simulink library "MSM_element"  (R2023b)
settings: Solver=VariableStepAuto  StartTime=0.0  StopTime=10.0  RelTol=1e-3
values from neighbouring files (symbols this model uses):
  A0 = msm_width * msm_height    (= 2.5e-06)    [MSM_mechanism_simulation_properties.m]    (also in MSM_simulation_data_processing.m = 4)
  constant_magnetic_stress = 3.27e+6    (= 3270000)    [MSM_mechanism_simulation_properties.m]
  contraction_initial = -msm_length * e_initial    (= -0.001)    [MSM_mechanism_simulation_properties.m]
  cos_a = cos(deg2rad(43.23))    [MSM_mechanism_simulation_properties.m]
  coulomb_friction_ts = 1e-10    [MSM_mechanism_simulation_properties.m]
  crystal_visualization_length = msm_length    (= 0.02)    [MSM_mechanism_simulation_properties.m]
  e_0 = 0.06    [MSM_mechanism_simulation_properties.m]
  k_0 = 11.8    [MSM_mechanism_simulation_properties.m]
  msm_height = 1e-3    (= 0.001)    [MSM_mechanism_simulation_properties.m]
  msm_length = 20e-3    (= 0.02)    [MSM_mechanism_simulation_properties.m]
  msm_mass = ro * A0 * msm_length    (= 0.0004)    [MSM_mechanism_simulation_properties.m]
  msm_width = 2.5e-3    (= 0.0025)    [MSM_mechanism_simulation_properties.m]    (also in model_validation.m = 0.001)
  one_side_absolute_offset = one_side_elongation_capacity * msm_length    (= 0.0001)    [MSM_mechanism_simulation_properties.m]
  ro = 8000    [MSM_mechanism_simulation_properties.m]
  tooth_pitch = tooth_pitch * tooth_size_modifier    (= 0.00039)    [MSM_mechanism_simulation_properties.m]    (also in get_tooth_properties.m = 0.00024661; msm_sim_runs_for_pid.m = evalin('base','tooth_pitch'); save_sim_result.m = evalin('base','tooth_pitch'))
  tooth_plate_height = 4.64e-3    (= 0.00464)    [MSM_mechanism_simulation_properties.m]
  Z = griddata(x,y,z,X,Y)    [MSM_simulation_data_processing.m]
undefined symbols (not defined in the file or in its folder): X, Y
libraries: sm_lib x14, nesl_utility x7, fl_lib x4
settings Model: Creator=h19343  LastModifiedBy=h19343
settings OptimizationCC: ReuseModelBlockBuffer=off

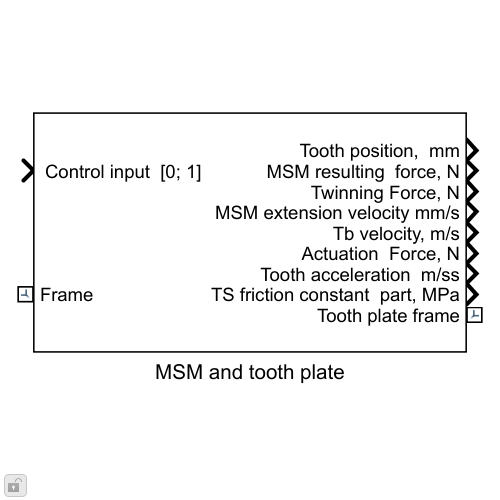
[thumbnail: Simulink's stored preview of the top-level diagram]
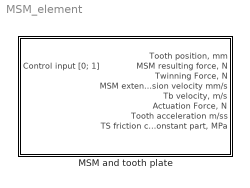
== system MSM_element ==
  MSM and tooth plate : Subsystem  mask{PositionTargetValue=contraction_initial}
      mask prompts: PositionTargetValue "ToothInitialPosition"
      mask TypeOptions PositionTargetValue: /PositionTargetValue

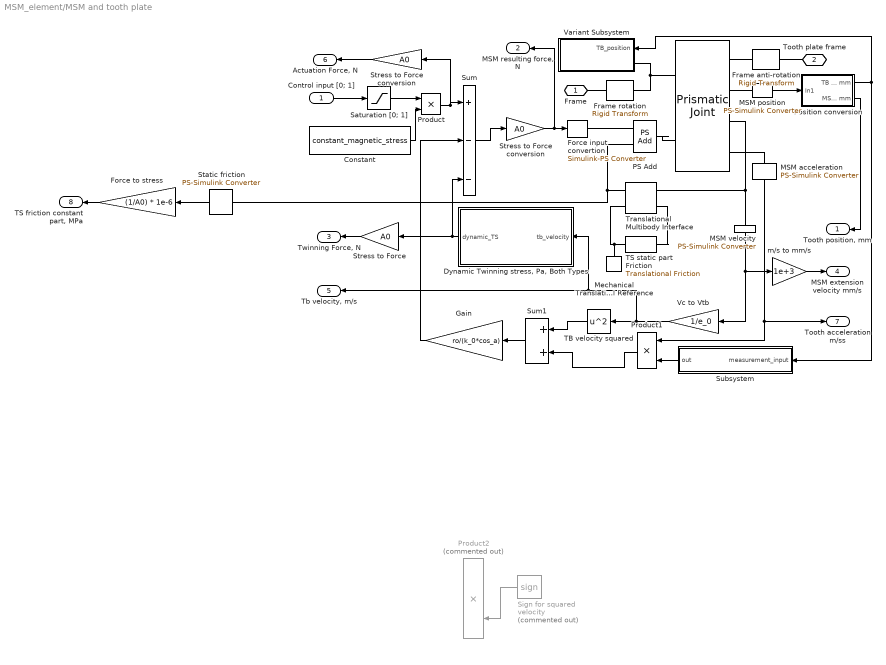
== system MSM_element/MSM and tooth plate ==
  " Control input [0; 1]" : Inport
  "   " : sm_lib/Joints/Prismatic Joint  JointMode=Normal  SenseConstraintForce=off  SenseConstraintForceX=off  SenseConstraintForceY=off  SenseConstraintForceZ=off  SenseConstraintTorque=off  SenseConstraintTorqueX=off  SenseConstraintTorqueY=off  SenseConstraintTorqueZ=off  SenseTotalForce=off  SenseTotalForceX=off  SenseTotalForceY=off  SenseTotalForceZ=off  SenseTotalTorque=off  SenseTotalTorqueX=off  SenseTotalTorqueY=off  SenseTotalTorqueZ=off  CompositeWrenchDir=FollowerOnBase  CompositeWrenchFrame=BaseFrame  EquilibriumPosition=0  EquilibriumPositionUnits=m  SpringStiffness=0  SpringStiffnessUnits=N/m  DampingCoefficient=bronze_steel_kinetic_friction  DampingCoefficientUnits=N/(m/s)  TorqueActuationMode=InputTorque  MotionActuationMode=ComputedMotion  SensePosition=on  SenseVelocity=on  SenseAcceleration=on  SenseTorqueForce=off  SenseLowerLimitTorqueForce=off  SenseUpperLimitTorqueForce=off  LowerLimitSpecify=on  LowerLimitBound=min_tooth_motion_range  LowerLimitBoundUnits=m  LowerLimitStiffness=1e6  LowerLimitStiffnessUnits=N/m  LowerLimitDamping=1e3  LowerLimitDampingUnits=N/(m/s)  LowerLimitTransitionRegionWidth=1e-4  LowerLimitTransitionRegionWidthUnits=m  UpperLimitSpecify=on  UpperLimitBound=max_tooth_motion_range  UpperLimitBoundUnits=m  UpperLimitStiffness=1e12  UpperLimitStiffnessUnits=N/m  UpperLimitDamping=1e4  UpperLimitDampingUnits=N/(m/s)  UpperLimitTransitionRegionWidth=1e-4  UpperLimitTransitionRegionWidthUnits=m  PositionTargetSpecify=on  PositionTargetPriority=Low  PositionTargetValue=PositionTargetValue  PositionTargetValueUnits=m  VelocityTargetSpecify=off  VelocityTargetPriority=High  VelocityTargetValue=0  VelocityTargetValueUnits=m/s
  Constant : Constant  Value=constant_magnetic_stress
  "Dynamic Twinning stress, Pa, Both Types" : MATLAB Function  TreatAsAtomicUnit=on
  Force input convertion : nesl_utility/Simulink-PS Converter  PhysicalDomain=network_engine_domain  SubClassName=ps_input  LeftPortType=input  RightPortType=output  PseudoPeriodic=off  Frequencies=[]  NoiseDistribution=none  NoiseParameters=[]  Unit=N  AffineConversion=off  FilteringAndDerivatives=filter  SimscapeFilterOrder=2  InputFilterTimeConstant=filter_time_constant  UdotUserProvided=0
  "Force to stress  " : Gain  Gain=(1/A0) * 1e-6
  Frame anti-rotation : sm_lib/Frames and Transforms/Rigid Transform  TranslationMethod=None  TranslationStandardOffset=0  TranslationStandardOffsetUnits=m  TranslationStandardAxis=+Z  TranslationCartesianOffset=[0 0 0]  TranslationCartesianOffsetUnits=m  TranslationROffset=0  TranslationROffsetUnits=m  TranslationZOffset=0  TranslationZOffsetUnits=m  TranslationThetaOffset=0  TranslationThetaOffsetUnits=deg  RotationMethod=StandardAxis  RotationAngleUnits=deg  RotationStandardAxis=-X  RotationAngle=-90  RotationArbitraryAxis=[0 0 1]  FollAlignAxisA=+X  BaseAlignAxisA=+Y  FollAlignAxisB=+Y  BaseAlignAxisB=+Z  RotationSequenceAxes=FollowerAxes  RotationSequence=XYX  RotationSequenceAngles=[0 0 0]  RotationSequenceAnglesUnits=deg  RotationMatrix=[1 0 0; 0 1 0; 0 0 1]  Quaternion=[1 0 0 0]
  Frame rotation : sm_lib/Frames and Transforms/Rigid Transform  TranslationMethod=None  TranslationStandardOffset=0  TranslationStandardOffsetUnits=m  TranslationStandardAxis=+Z  TranslationCartesianOffset=[0 0 0]  TranslationCartesianOffsetUnits=m  TranslationROffset=0  TranslationROffsetUnits=m  TranslationZOffset=0  TranslationZOffsetUnits=m  TranslationThetaOffset=0  TranslationThetaOffsetUnits=deg  RotationMethod=StandardAxis  RotationAngleUnits=deg  RotationStandardAxis=-X  RotationAngle=90  RotationArbitraryAxis=[0 0 1]  FollAlignAxisA=+X  BaseAlignAxisA=+Y  FollAlignAxisB=+Y  BaseAlignAxisB=+Z  RotationSequenceAxes=FollowerAxes  RotationSequence=XYX  RotationSequenceAngles=[0 0 0]  RotationSequenceAnglesUnits=deg  RotationMatrix=[1 0 0; 0 1 0; 0 0 1]  Quaternion=[1 0 0 0]
  Gain : Gain  Gain=ro/(k_0*cos_a)
  MSM acceleration : nesl_utility/PS-Simulink Converter  PhysicalDomain=network_engine_domain  SubClassName=ps_output  LeftPortType=input  RightPortType=output  PseudoPeriodic=off  Frequencies=[]  VectorFormat=inherit  Unit=inherit  AffineConversion=off
  MSM velocity : nesl_utility/PS-Simulink Converter  PhysicalDomain=network_engine_domain  SubClassName=ps_output  LeftPortType=input  RightPortType=output  PseudoPeriodic=off  Frequencies=[]  VectorFormat=inherit  Unit=inherit  AffineConversion=off
  MSM position : nesl_utility/PS-Simulink Converter  PhysicalDomain=network_engine_domain  SubClassName=ps_output  LeftPortType=input  RightPortType=output  PseudoPeriodic=off  Frequencies=[]  VectorFormat=inherit  Unit=inherit  AffineConversion=off
  Mechanical Translational Reference : fl_lib/Mechanical/Translational Elements/Mechanical Translational Reference
  PS Add : fl_lib/Physical Signals/Functions/PS Add
  Position conversion : Subsystem
  Product : Product
  Product1 : Product
  Product2 : Product  Commented=on
  Saturation [0; 1] : Saturate  UpperLimit=1  LowerLimit=0
  Sign for squared velocity : Signum  Commented=on
  Static friction : nesl_utility/PS-Simulink Converter  PhysicalDomain=network_engine_domain  SubClassName=ps_output  LeftPortType=input  RightPortType=output  PseudoPeriodic=off  Frequencies=[]  VectorFormat=inherit  Unit=inherit  AffineConversion=off
  Stress to Force : Gain  Gain=A0
  Stress to Force conversion : Gain  Gain=A0
  "Stress to Force conversion   " : Gain  Gain=A0
  Subsystem : Subsystem
      mask Display:
      | text(0.05,0.5,'{out =}  m_0 / ( \rho * A_0 ) + L - L_0',...
      | HorizontalAlignment = 'left',texmode = 'on')
  Sum : Sum  Inputs=+--
  Sum1 : Sum
  TB velocity squared : Math  Operator=square
  TS static part Friction : fl_lib/Mechanical/Translational Elements/Translational Friction  brkwy_frc=coulomb_friction_ts * (1 + 1e-5) N  brkwy_vel=1e-5 m/s  Col_frc=coulomb_friction_ts N  visc_coef=0 N*s/m  v_specify=off  v_priority=None  v=0 m/s  v_nominal_specify=off  v_nominal_unit=m/s  v_nominal_value=1  f_specify=off  f_priority=None  f=0 N  f_nominal_specify=off  f_nominal_unit=N  f_nominal_value=1
      settings: InternalSimscapePortConfiguration="{\"Bottom\":[],\"Left\":[{\"id\":\"R\",\"label\":\"R\",\"type\":\"foundation.mechanical.translational.translational\"}],\"Right\":[{\"id\":\"C\",\"label\":\"C\",\"type\":\"foundation.mechanical.translational.translational\"}],\"Top\":[]}"
  Translational Multibody Interface : fl_lib/Mechanical/Multibody Interfaces/Translational Multibody Interface
  Variant Subsystem : Subsystem  InitFcn=|  Variant=on
      | simple_visuals_variant = Simulink.Variant('simplified_visualization == true');
      | full_visuals_variant = Simulink.Variant('simplified_visualization == false');
      settings: PortSchema="{\"entries\":[{\"content\":{\"sides\":[{\"content\":{\"connectorIds\":[\"LConn1\",\"In1\"]},\"type\":\"ConnectorPlacement.EquallySpacedRectSide\",\"uuid\":\"521faf6a-dace-4634-9239-1a534469285d\"},{\"content\":{\"side\":\"RIGHT\"},\"type\":\"ConnectorPlacement.EquallySpacedRectSide\",\"uuid\":\"3bf57a7f-6223-4aa5-b9ce-2577a1bef6cc\"},{\"content\":{\"side\":\"TOP\"},\"type\":\"ConnectorPlacement.EquallySpacedRectSide\",\"uuid\":\"83854e2c-9733-4a76-abdf-07b6192acd72\"}]},\"type\":\"ConnectorPlacement.EquallySpacedConnector\",\"uuid\":\"3009cfd0-5b5f-49c0-93d8-2e0b9647e6c0\"}],\"packageUris\":[\"http://schema.mathworks.com/mf0/Connector/R2020b\"],\"version\":\"1.0\"}"
      mask Display:
      | text(0.05,0.65,'TB position',...
      | HorizontalAlignment = 'left',texmode = 'on')
      | text(0.05,0.35,'visualization block',...
      | HorizontalAlignment = 'left',texmode = 'on')
  Vc to Vtb : Gain  Gain=1/e_0
  m/s to mm/s : Gain  Gain=1e+3
  Frame : PMIOPort  Side=Left
  Tooth plate frame : PMIOPort  Port=2  Side=Right
  "Tooth position, mm" : Outport
  "      MSM resulting force, N" : Outport  Port=2
  "Twinning Force, N" : Outport  Port=3
  MSM extension velocity mm/s : Outport  Port=4
  "Tb velocity, m/s" : Outport  Port=5
  "Actuation Force, N" : Outport  Port=6
  Tooth acceleration m/ss : Outport  Port=7
  "TS friction constant part, MPa" : Outport  Port=8
  wires:
  " Control input [0; 1]"/1 -> Saturation [0; 1]/1
  Saturation [0; 1]/1 -> Product/1
  Constant/1 -> Product/2
  Stress to Force conversion/1 -> "      MSM resulting force, N"/1, Force input convertion/1
  Sum/1 -> Stress to Force conversion/1
  Product/1 -> Sum/1, "Stress to Force conversion   "/1
  Stress to Force/1 -> "Twinning Force, N"/1
  "Stress to Force conversion   "/1 -> "Actuation Force, N"/1
  MSM velocity/1 -> Vc to Vtb/1, m/s to mm/s/1
  "Dynamic Twinning stress, Pa, Both Types"/1(dynamic_TS) -> Sum/3, Stress to Force/1
  MSM acceleration/1 -> Tooth acceleration m/ss/1, Product1/1
  Sum1/1 -> Gain/1
  Product1/1 -> Sum1/2
  Sign for squared velocity/1 -> Product2/2
  Vc to Vtb/1 -> "Dynamic Twinning stress, Pa, Both Types"/1(tb_velocity), "Tb velocity, m/s"/1, TB velocity squared/1
  m/s to mm/s/1 -> MSM extension velocity mm/s/1
  "Force to stress  "/1 -> "TS friction constant part, MPa"/1
  TB velocity squared/1 -> Sum1/1
  Gain/1 -> Sum/2
  Subsystem/1(out) -> Product1/2
  Position conversion/1("TB pos, mm") -> Variant Subsystem/1(TB_position), Subsystem/1(measurement_input)
  MSM position/1 -> Position conversion/1(In1)
  Position conversion/2("MSM pos, mm") -> "Tooth position, mm"/1
  Static friction/1 -> "Force to stress  "/1
  connections:
  Tooth plate frame/RConn1 -- Frame anti-rotation/RConn1
  MSM position/LConn1 -- "   "/RConn2
  Frame anti-rotation/LConn1 -- "   "/RConn1
  "   "/LConn1 -- Frame rotation/RConn1 -- Variant Subsystem/LConn1
  Frame rotation/LConn1 -- Frame/RConn1
  Translational Multibody Interface/RConn1 -- MSM velocity/LConn1 -- "   "/RConn3
  MSM acceleration/LConn1 -- "   "/RConn4
  PS Add/LConn2 -- Translational Multibody Interface/LConn1 -- Static friction/LConn1
  Mechanical Translational Reference/LConn1 -- Translational Multibody Interface/LConn2 -- TS static part Friction/RConn1
  TS static part Friction/LConn1 -- Translational Multibody Interface/RConn2
  Force input convertion/RConn1 -- PS Add/LConn1
  PS Add/RConn1 -- "   "/LConn2

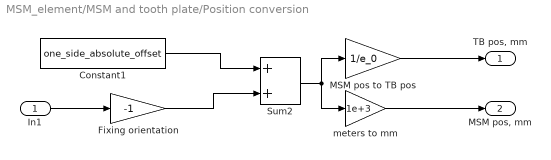
== system MSM_element/MSM and tooth plate/Position conversion ==
  In1 : Inport
  Constant1 : Constant  Value=one_side_absolute_offset
  Fixing orientation : Gain  Gain=-1
  MSM pos to TB pos : Gain  Gain=1/e_0
  Sum2 : Sum
  meters to mm : Gain  Gain=1e+3
  "TB pos, mm" : Outport
  "MSM pos, mm" : Outport  Port=2
  wires:
  Fixing orientation/1 -> Sum2/2
  Sum2/1 -> MSM pos to TB pos/1, meters to mm/1
  meters to mm/1 -> "MSM pos, mm"/1
  Constant1/1 -> Sum2/1
  In1/1 -> Fixing orientation/1
  MSM pos to TB pos/1 -> "TB pos, mm"/1

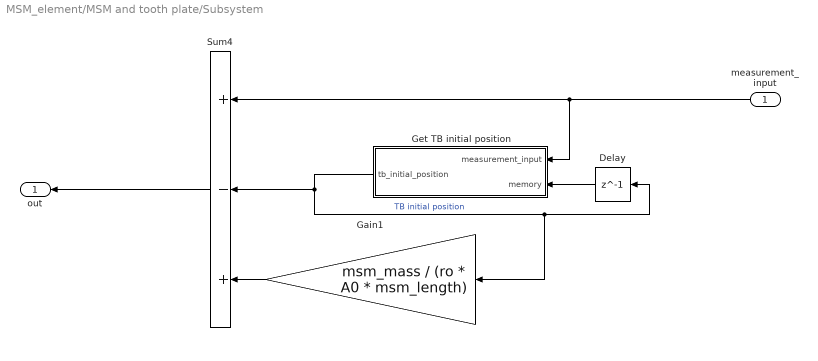
== system MSM_element/MSM and tooth plate/Subsystem ==
  measurement_input : Inport
  Delay : Delay  DelayLength=1  InitialCondition=-1
  Gain1 : Gain  Gain=msm_mass / (ro * A0 * msm_length)
  Get TB initial position : MATLAB Function  TreatAsAtomicUnit=on
  Sum4 : Sum  Inputs=+-+
  out : Outport
  wires:
  Get TB initial position/1(tb_initial_position) -> Gain1/1, Delay/1, Sum4/2  "TB initial position"
  Gain1/1 -> Sum4/3
  Delay/1 -> Get TB initial position/2(memory)
  measurement_input/1 -> Sum4/1, Get TB initial position/1(measurement_input)
  Sum4/1 -> out/1

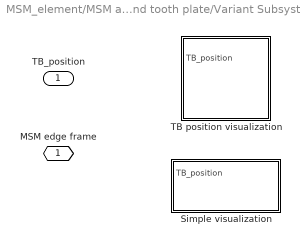
== system MSM_element/MSM and tooth plate/Variant Subsystem ==
  TB_position : Inport
  Simple visualization : Subsystem  VariantControl=simple_visuals_variant
  TB position visualization : Subsystem  AncestorBlock=MSM_element_08_04_2024/MSM and tooth plate/TB position visualization  VariantControl=full_visuals_variant
  MSM edge frame : PMIOPort  Side=Left

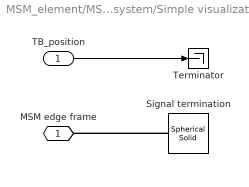
== system MSM_element/MSM and tooth plate/Variant Subsystem/Simple visualization ==
  TB_position : Inport
  Signal termination : sm_lib/Body Elements/Spherical Solid  GraphicAmbientColor=[0.15 0.15 0.15 1.0]  BasedOnType=Mass  CenterOfMass=[0 0 0]  CenterOfMassUnits=m  GraphicDiffuseColor=[0.5 0.5 0.5]  Density=1000  DensityUnits=kg/m^3  DoExposeReferenceFrame=on  GraphicEmissiveColor=[0.0 0.0 0.0 1.0]  ExportEntireGeometry=off  SerializedExposedGeometries=<ExposedGeometries/>  SerializedFrames=<Frames/>  MarkerShape=Sphere  MarkerSize=10  GraphicType=None  InertiaType=CalculateFromGeometry  Mass=1e-12  MassUnits=kg  MomentsOfInertia=[1 1 1]  MomentsOfInertiaUnits=kg*m^2  GraphicOpacity=1.0  ProductsOfInertia=[0 0 0]  ProductsOfInertiaUnits=kg*m^2  GraphicShininess=75  GraphicSpecularColor=[0.5 0.5 0.5 1.0]  SphereRadius=1  SphereRadiusUnits=m  GraphicVisPropType=SimpleVisualProperties
  Terminator : Terminator
  MSM edge frame : PMIOPort  Side=Left
  wires:
  TB_position/1 -> Terminator/1
  connections:
  Signal termination/RConn1 -- MSM edge frame/RConn1

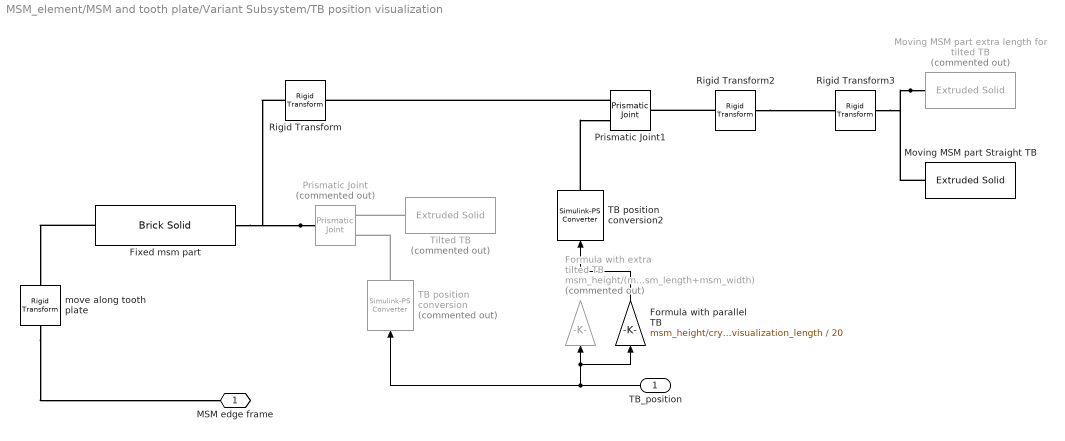
== system MSM_element/MSM and tooth plate/Variant Subsystem/TB position visualization ==
  TB_position : Inport
  Fixed msm part : sm_lib/Body Elements/Brick Solid  GraphicAmbientColor=[0.15 0.15 0.15 1.0]  BasedOnType=Mass  BrickDimensions=[msm_width msm_height crystal_visualization_length]  BrickDimensionsUnits=m  CenterOfMass=[0 0 0]  CenterOfMassUnits=m  GraphicDiffuseColor=[0.6 0.6 0.6]  Density=1000  DensityUnits=kg/m^3  DoExposeReferenceFrame=off  GraphicEmissiveColor=[0.0 0.0 0.0 1.0]  ExportEntireGeometry=off  SerializedFrames=<Frames><Frame><Id>Frame1</Id><Value><Name>End frame</Name><Origin><Source>GeometricFeature</Source><FeatureName>-z surface</FeatureName></Origin><PrimaryAxis><DefinedDirection>+Z</DefinedDirection><Source>ReferenceFrame</Source><SourceDirection>-Z</SourceDirection><FeatureName></FeatureName></PrimaryAxis><SecondaryAxis><DefinedDirection>+X</DefinedDirection><Source>ReferenceFrame</Source><SourceDirection>+X</SourceDirection><FeatureName></FeatureName></SecondaryAxis></Value></Frame><Frame><Id>Frame2</Id><Value><Name>End rotation</Name><Origin><Source>GeometricFeature</Source><FeatureName>+y -z curve</FeatureName></Origin><PrimaryAxis><DefinedDirection>+Z</DefinedDirection><Source>ReferenceFrame</Source><SourceDirection>-Z</SourceDirection><FeatureName></FeatureName></PrimaryAxis><SecondaryAxis><DefinedDirection>+X</DefinedDirection><Source>ReferenceFrame</Source><SourceDirection>+X</SourceDirection><FeatureName></FeatureName></SecondaryAxis></Value></Frame></Frames>  MarkerShape=Sphere  MarkerSize=10  GraphicType=FromGeometry  InertiaType=CalculateFromGeometry  Mass=1e-12  MassUnits=kg  MomentsOfInertia=[1 1 1]  MomentsOfInertiaUnits=kg*m^2  GraphicOpacity=1.0  ProductsOfInertia=[0 0 0]  ProductsOfInertiaUnits=kg*m^2  GraphicShininess=75  GraphicSpecularColor=[0.5 0.5 0.5 1.0]  GraphicVisPropType=SimpleVisualProperties
  Formula with extra tilted TB : Gain  Commented=on  Gain=msm_height/(msm_length+msm_width)
  Formula with parallel TB : Gain  Gain=msm_height/crystal_visualization_length / 20
  Moving MSM part Straight TB : sm_lib/Body Elements/Extruded Solid  GraphicAmbientColor=[0.15 0.15 0.15 1.0]  BasedOnType=Mass  CenterOfMass=[0 0 0]  CenterOfMassUnits=m  GraphicDiffuseColor=moving_tb_color  ExportConvexHullGeometry=off  ExtrusionCrossSection=[crystal_visualization_length msm_height / 20; 0 msm_height / 20; 0 0]  ExtrusionCrossSectionUnits=m  Density=1000  DensityUnits=kg/m^3  DoExposeReferenceFrame=on  GraphicEmissiveColor=[0.0 0.0 0.0 1.0]  ExportEntireGeometry=off  ExtrusionLength=msm_width  ExtrusionLengthUnits=m  ExtrusionType=General  SerializedFrames=<Frames/>  MarkerShape=Sphere  MarkerSize=10  GraphicType=FromGeometry  InertiaType=CalculateFromGeometry  Mass=1e-12  MassUnits=kg  MomentsOfInertia=[1 1 1]  MomentsOfInertiaUnits=kg*m^2  PolygonNumSides=3  GraphicOpacity=1.0  PolygonOuterRadius=1  PolygonOuterRadiusUnits=m  ProductsOfInertia=[0 0 0]  ProductsOfInertiaUnits=kg*m^2  GraphicShininess=75  GraphicSpecularColor=[0.5 0.5 0.5 1.0]  GraphicVisPropType=SimpleVisualProperties
  Moving MSM part extra length for tilted TB : sm_lib/Body Elements/Extruded Solid  Commented=on  GraphicAmbientColor=[0.15 0.15 0.15 1.0]  BasedOnType=Mass  CenterOfMass=[0 0 0]  CenterOfMassUnits=m  GraphicDiffuseColor=moving_tb_color  ExportConvexHullGeometry=off  ExtrusionCrossSection=[msm_length+msm_width msm_height; 0 msm_height; 0 0]  ExtrusionCrossSectionUnits=m  Density=1000  DensityUnits=kg/m^3  DoExposeReferenceFrame=on  GraphicEmissiveColor=[0.0 0.0 0.0 1.0]  ExportEntireGeometry=off  ExtrusionLength=msm_width  ExtrusionLengthUnits=m  ExtrusionType=General  SerializedFrames=<Frames/>  MarkerShape=Sphere  MarkerSize=10  GraphicType=FromGeometry  InertiaType=CalculateFromGeometry  Mass=1e-12  MassUnits=kg  MomentsOfInertia=[1 1 1]  MomentsOfInertiaUnits=kg*m^2  PolygonNumSides=3  GraphicOpacity=1.0  PolygonOuterRadius=1  PolygonOuterRadiusUnits=m  ProductsOfInertia=[0 0 0]  ProductsOfInertiaUnits=kg*m^2  GraphicShininess=75  GraphicSpecularColor=[0.5 0.5 0.5 1.0]  GraphicVisPropType=SimpleVisualProperties
  Prismatic Joint : sm_lib/Joints/Prismatic Joint  Commented=on  JointMode=Normal  SenseConstraintForce=off  SenseConstraintForceX=off  SenseConstraintForceY=off  SenseConstraintForceZ=off  SenseConstraintTorque=off  SenseConstraintTorqueX=off  SenseConstraintTorqueY=off  SenseConstraintTorqueZ=off  SenseTotalForce=off  SenseTotalForceX=off  SenseTotalForceY=off  SenseTotalForceZ=off  SenseTotalTorque=off  SenseTotalTorqueX=off  SenseTotalTorqueY=off  SenseTotalTorqueZ=off  CompositeWrenchDir=FollowerOnBase  CompositeWrenchFrame=BaseFrame  EquilibriumPosition=0  EquilibriumPositionUnits=m  SpringStiffness=0  SpringStiffnessUnits=N/m  DampingCoefficient=0  DampingCoefficientUnits=N/(m/s)  TorqueActuationMode=ComputedTorque  MotionActuationMode=InputMotion  SensePosition=off  SenseVelocity=off  SenseAcceleration=off  SenseTorqueForce=off  SenseLowerLimitTorqueForce=off  SenseUpperLimitTorqueForce=off  LowerLimitSpecify=off  LowerLimitBound=-1  LowerLimitBoundUnits=m  LowerLimitStiffness=1e6  LowerLimitStiffnessUnits=N/m  LowerLimitDamping=1e3  LowerLimitDampingUnits=N/(m/s)  LowerLimitTransitionRegionWidth=1e-4  LowerLimitTransitionRegionWidthUnits=m  UpperLimitSpecify=off  UpperLimitBound=1  UpperLimitBoundUnits=m  UpperLimitStiffness=1e6  UpperLimitStiffnessUnits=N/m  UpperLimitDamping=1e3  UpperLimitDampingUnits=N/(m/s)  UpperLimitTransitionRegionWidth=1e-4  UpperLimitTransitionRegionWidthUnits=m  PositionTargetSpecify=off  PositionTargetPriority=High  PositionTargetValue=0  PositionTargetValueUnits=m  VelocityTargetSpecify=off  VelocityTargetPriority=High  VelocityTargetValue=0  VelocityTargetValueUnits=m/s
  Prismatic Joint1 : sm_lib/Joints/Prismatic Joint  JointMode=Normal  SenseConstraintForce=off  SenseConstraintForceX=off  SenseConstraintForceY=off  SenseConstraintForceZ=off  SenseConstraintTorque=off  SenseConstraintTorqueX=off  SenseConstraintTorqueY=off  SenseConstraintTorqueZ=off  SenseTotalForce=off  SenseTotalForceX=off  SenseTotalForceY=off  SenseTotalForceZ=off  SenseTotalTorque=off  SenseTotalTorqueX=off  SenseTotalTorqueY=off  SenseTotalTorqueZ=off  CompositeWrenchDir=FollowerOnBase  CompositeWrenchFrame=BaseFrame  EquilibriumPosition=0  EquilibriumPositionUnits=m  SpringStiffness=0  SpringStiffnessUnits=N/m  DampingCoefficient=0  DampingCoefficientUnits=N/(m/s)  TorqueActuationMode=ComputedTorque  MotionActuationMode=InputMotion  SensePosition=off  SenseVelocity=off  SenseAcceleration=off  SenseTorqueForce=off  SenseLowerLimitTorqueForce=off  SenseUpperLimitTorqueForce=off  LowerLimitSpecify=off  LowerLimitBound=-1  LowerLimitBoundUnits=m  LowerLimitStiffness=1e6  LowerLimitStiffnessUnits=N/m  LowerLimitDamping=1e3  LowerLimitDampingUnits=N/(m/s)  LowerLimitTransitionRegionWidth=1e-4  LowerLimitTransitionRegionWidthUnits=m  UpperLimitSpecify=off  UpperLimitBound=1  UpperLimitBoundUnits=m  UpperLimitStiffness=1e6  UpperLimitStiffnessUnits=N/m  UpperLimitDamping=1e3  UpperLimitDampingUnits=N/(m/s)  UpperLimitTransitionRegionWidth=1e-4  UpperLimitTransitionRegionWidthUnits=m  PositionTargetSpecify=off  PositionTargetPriority=High  PositionTargetValue=0  PositionTargetValueUnits=m  VelocityTargetSpecify=off  VelocityTargetPriority=High  VelocityTargetValue=0  VelocityTargetValueUnits=m/s
  Rigid Transform : sm_lib/Frames and Transforms/Rigid Transform  TranslationMethod=None  TranslationStandardOffset=0  TranslationStandardOffsetUnits=m  TranslationStandardAxis=+Z  TranslationCartesianOffset=[0 0 0]  TranslationCartesianOffsetUnits=m  TranslationROffset=0  TranslationROffsetUnits=m  TranslationZOffset=0  TranslationZOffsetUnits=m  TranslationThetaOffset=0  TranslationThetaOffsetUnits=deg  RotationMethod=StandardAxis  RotationAngleUnits=deg  RotationStandardAxis=+X  RotationAngle=90  RotationArbitraryAxis=[0 0 1]  FollAlignAxisA=+X  BaseAlignAxisA=+Y  FollAlignAxisB=+Y  BaseAlignAxisB=+Z  RotationSequenceAxes=FollowerAxes  RotationSequence=XYX  RotationSequenceAngles=[0 0 0]  RotationSequenceAnglesUnits=deg  RotationMatrix=[1 0 0; 0 1 0; 0 0 1]  Quaternion=[1 0 0 0]
  Rigid Transform2 : sm_lib/Frames and Transforms/Rigid Transform  TranslationMethod=None  TranslationStandardOffset=0  TranslationStandardOffsetUnits=m  TranslationStandardAxis=+Z  TranslationCartesianOffset=[0 0 0]  TranslationCartesianOffsetUnits=m  TranslationROffset=0  TranslationROffsetUnits=m  TranslationZOffset=0  TranslationZOffsetUnits=m  TranslationThetaOffset=0  TranslationThetaOffsetUnits=deg  RotationMethod=StandardAxis  RotationAngleUnits=deg  RotationStandardAxis=+X  RotationAngle=90  RotationArbitraryAxis=[0 0 1]  FollAlignAxisA=+X  BaseAlignAxisA=+Y  FollAlignAxisB=+Y  BaseAlignAxisB=+Z  RotationSequenceAxes=FollowerAxes  RotationSequence=XYX  RotationSequenceAngles=[0 0 0]  RotationSequenceAnglesUnits=deg  RotationMatrix=[1 0 0; 0 1 0; 0 0 1]  Quaternion=[1 0 0 0]
  Rigid Transform3 : sm_lib/Frames and Transforms/Rigid Transform  TranslationMethod=None  TranslationStandardOffset=0  TranslationStandardOffsetUnits=m  TranslationStandardAxis=+Z  TranslationCartesianOffset=[0 0 0]  TranslationCartesianOffsetUnits=m  TranslationROffset=0  TranslationROffsetUnits=m  TranslationZOffset=0  TranslationZOffsetUnits=m  TranslationThetaOffset=0  TranslationThetaOffsetUnits=deg  RotationMethod=StandardAxis  RotationAngleUnits=deg  RotationStandardAxis=-Y  RotationAngle=90  RotationArbitraryAxis=[0 0 1]  FollAlignAxisA=+X  BaseAlignAxisA=+Y  FollAlignAxisB=+Y  BaseAlignAxisB=+Z  RotationSequenceAxes=FollowerAxes  RotationSequence=XYX  RotationSequenceAngles=[0 0 0]  RotationSequenceAnglesUnits=deg  RotationMatrix=[1 0 0; 0 1 0; 0 0 1]  Quaternion=[1 0 0 0]
  TB position conversion : nesl_utility/Simulink-PS Converter  Commented=on  PhysicalDomain=network_engine_domain  SubClassName=ps_input  LeftPortType=input  RightPortType=output  PseudoPeriodic=off  Frequencies=[]  NoiseDistribution=none  NoiseParameters=[]  Unit=m  AffineConversion=off  FilteringAndDerivatives=filter  SimscapeFilterOrder=2  InputFilterTimeConstant=filter_time_constant  UdotUserProvided=0
  TB position conversion2 : nesl_utility/Simulink-PS Converter  PhysicalDomain=network_engine_domain  SubClassName=ps_input  LeftPortType=input  RightPortType=output  PseudoPeriodic=off  Frequencies=[]  NoiseDistribution=none  NoiseParameters=[]  Unit=m  AffineConversion=off  FilteringAndDerivatives=filter  SimscapeFilterOrder=2  InputFilterTimeConstant=filter_time_constant  UdotUserProvided=0
  Tilted TB : sm_lib/Body Elements/Extruded Solid  Commented=on  GraphicAmbientColor=[0.15 0.15 0.15 1.0]  BasedOnType=Mass  CenterOfMass=[0 0 0]  CenterOfMassUnits=m  GraphicDiffuseColor=moving_tb_color  ExportConvexHullGeometry=off  ExtrusionCrossSection=[msm_width msm_width; 0 msm_width; 0 0]  ExtrusionCrossSectionUnits=m  Density=1000  DensityUnits=kg/m^3  DoExposeReferenceFrame=off  GraphicEmissiveColor=[0.0 0.0 0.0 1.0]  ExportEntireGeometry=off  ExtrusionLength=msm_height / 10  ExtrusionLengthUnits=m  ExtrusionType=General  SerializedFrames=<Frames><Frame><Id>Frame1</Id><Value><Name>Sliding frame</Name><Origin><Source>GeometricFeature</Source><FeatureName>side surface 1</FeatureName></Origin><PrimaryAxis><DefinedDirection>+Z</DefinedDirection><Source>ReferenceFrame</Source><SourceDirection>+Y</SourceDirection><FeatureName></FeatureName></PrimaryAxis><SecondaryAxis><DefinedDirection>+X</DefinedDirection><Source>ReferenceFrame</Source><SourceDirection>+X</SourceDirection><FeatureName></FeatureName></SecondaryAxis></Value></Frame></Frames>  MarkerShape=Sphere  MarkerSize=10  GraphicType=FromGeometry  InertiaType=CalculateFromGeometry  Mass=1e-12  MassUnits=kg  MomentsOfInertia=[1 1 1]  MomentsOfInertiaUnits=kg*m^2  PolygonNumSides=3  GraphicOpacity=1.0  PolygonOuterRadius=1  PolygonOuterRadiusUnits=m  ProductsOfInertia=[0 0 0]  ProductsOfInertiaUnits=kg*m^2  GraphicShininess=75  GraphicSpecularColor=[0.5 0.5 0.5 1.0]  GraphicVisPropType=SimpleVisualProperties
  move along tooth plate : sm_lib/Frames and Transforms/Rigid Transform  TranslationMethod=StandardAxis  TranslationStandardOffset=tooth_plate_height+tooth_pitch  TranslationStandardOffsetUnits=m  TranslationStandardAxis=+Z  TranslationCartesianOffset=[0 0 0]  TranslationCartesianOffsetUnits=m  TranslationROffset=0  TranslationROffsetUnits=m  TranslationZOffset=0  TranslationZOffsetUnits=m  TranslationThetaOffset=0  TranslationThetaOffsetUnits=deg  RotationMethod=None  RotationAngleUnits=deg  RotationStandardAxis=+Z  RotationAngle=0.0  RotationArbitraryAxis=[0 0 1]  FollAlignAxisA=+X  BaseAlignAxisA=+Y  FollAlignAxisB=+Y  BaseAlignAxisB=+Z  RotationSequenceAxes=FollowerAxes  RotationSequence=XYX  RotationSequenceAngles=[0 0 0]  RotationSequenceAnglesUnits=deg  RotationMatrix=[1 0 0; 0 1 0; 0 0 1]  Quaternion=[1 0 0 0]
  MSM edge frame : PMIOPort  Side=Left
  wires:
  Formula with parallel TB/1 -> TB position conversion2/1
  TB_position/1 -> Formula with extra tilted TB/1, Formula with parallel TB/1, TB position conversion/1
  connections:
  TB position conversion2/RConn1 -- Prismatic Joint1/LConn2
  TB position conversion/RConn1 -- Prismatic Joint/LConn2
  Moving MSM part extra length for tilted TB/RConn1 -- Moving MSM part Straight TB/RConn1 -- Rigid Transform3/LConn1
  Prismatic Joint1/LConn1 -- Rigid Transform/RConn1
  move along tooth plate/RConn1 -- MSM edge frame/RConn1
  Fixed msm part/LConn1 -- move along tooth plate/LConn1
  Rigid Transform2/LConn1 -- Rigid Transform3/RConn1
  Rigid Transform2/RConn1 -- Prismatic Joint1/RConn1
  Tilted TB/LConn1 -- Prismatic Joint/LConn1
  Prismatic Joint/RConn1 -- Rigid Transform/LConn1 -- Fixed msm part/RConn1

== matlab function MSM_element/MSM and tooth plate/Subsystem/Get TB initial position ==
  data: measurement_input input; tb_initial_position output; memory input
function tb_initial_position = fcn(measurement_input, memory)

if measurement_input < 0
    error("measured current TB position is less than zero. This error is for debugging only")
end

if memory < 0
    tb_initial_position = measurement_input;
else
    tb_initial_position = memory;
end

== matlab function MSM_element/MSM and tooth plate/Dynamic Twinning stress, Pa, Both Types ==
  data: tb_velocity input; dynamic_TS output; tb_type parameter
function dynamic_TS = fcn(tb_velocity,...
    tb_type) %,  is a parameter

% 0.1 +
if tb_type == 1
    dynamic_TS = 0.81*abs(tb_velocity) *...
        sign(tb_velocity) * (1e+6); % From Saren and Ullakko 2017
elseif tb_type == 2
    dynamic_TS = ( 0.014*power(abs(tb_velocity), 1.4)) *...
        sign(tb_velocity) * (1e+6); % From Saren and Ullakko 2017
else
    dynamic_TS = NaN;
end
% --- The following idea does not work as intended --- 
% quasi-static option
% if abs(tb_velocity) < 1e-6
%     dynamic_TS = -sign(resulting_force) * min([abs(dynamic_TS),abs(resulting_force)]);
% end
